simulink model "Sample5"  (Simulink 7.6)
settings: Solver=ode45  StartTime=0.0  StopTime=10.0  RelTol=1e-3
libraries: commdigbbndfm2 x2, dspbuff3 x1, simulink x1, commblkcod2 x1
settings Model: Creator=admin  LastModifiedBy=admin
settings OptimizationCC: InitFltsAndDblsToZero=on
settings DebuggingCC: SaveWithParameterizedLinksMsg=none  SignalResolutionControl=TryResolveAllWithWarning  MultiTaskDSMMsg=warning  MultiTaskCondExecSysMsg=none  StrictBusMsg=Warning
settings RTWCC: IncludeERTFirstTime=on
settings GRTTargetCC: TargetFcnLib=ansi_tfl_tmw.mat

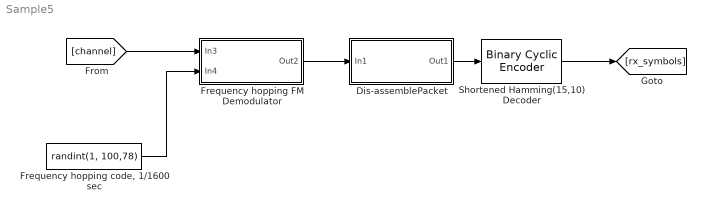
== system Sample5 ==
  Dis-assemblePacket : Subsystem
  Frequency hopping FM Demodulator : Subsystem
  "Frequency hopping code, 1/1600 sec" : FromWorkspace  VariableName=randint(1, 100,78)  SampleTime=1/1600
  Shortened Hamming(15,10) Decoder : commblkcod2/Binary Cyclic Encoder  SystemSampleTime=-1  n=15  p=[1 1 0 1 0 1]
  wires:
  [channel] -> Frequency hopping FM Demodulator/1(In3)
  "Frequency hopping code, 1/1600 sec"/1 -> Frequency hopping FM Demodulator/2(In4)
  Frequency hopping FM Demodulator/1(Out2) -> Dis-assemblePacket/1(In1)
  Dis-assemblePacket/1(Out1) -> Shortened Hamming(15,10) Decoder/1
  Shortened Hamming(15,10) Decoder/1 -> [rx_symbols]

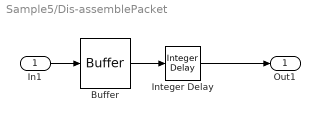
== system Sample5/Dis-assemblePacket ==
  In1 : Inport
  Buffer : dspbuff3/Buffer  N=15  V=0  ic=0
  Integer Delay : simulink/Discrete/Integer Delay  vinit=0.0  samptime=-1  NumDelays=10
  Out1 : Outport
  wires:
  In1/1 -> Buffer/1
  Buffer/1 -> Integer Delay/1
  Integer Delay/1 -> Out1/1

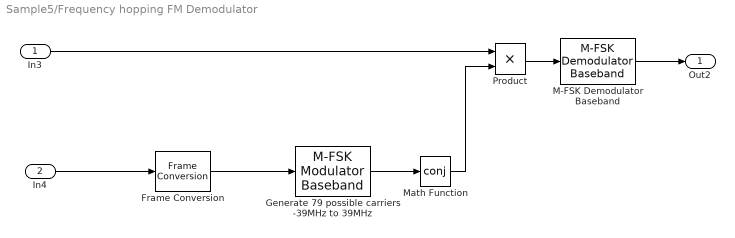
== system Sample5/Frequency hopping FM Demodulator ==
  In3 : Inport
  In4 : Inport  Port=2
  Frame Conversion : FrameConversion
  Generate 79 possible carriers -39MHz to 39MHz : commdigbbndfm2/M-FSK Modulator Baseband  M=19  InType=Integer  Enc=Binary  freqSep=1e6  phaseType=Continuous  numSamp=6.25e4  outDataType=double
  M-FSK Demodulator Baseband : commdigbbndfm2/M-FSK Demodulator Baseband  M=2  OutType=Integer  Dec=Binary  freqSep=10  numSamp=100  outDataType=double
  Math Function : Math  Operator=conj  SaturateOnIntegerOverflow=on
  Product : Product  RndMeth=Zero
  Out2 : Outport
  wires:
  In3/1 -> Product/1
  Frame Conversion/1 -> Generate 79 possible carriers -39MHz to 39MHz/1
  In4/1 -> Frame Conversion/1
  Generate 79 possible carriers -39MHz to 39MHz/1 -> Math Function/1
  Math Function/1 -> Product/2
  Product/1 -> M-FSK Demodulator Baseband/1
  M-FSK Demodulator Baseband/1 -> Out2/1
